simulink model "bh_SM_quad_and_PEND_ORIG"  (R2020a)
settings: Solver=ode23t  StartTime=0.0  StopTime=200  FixedStep=0.001  RelTol=1e-5  EnableMultiTasking=on
undefined symbols (not defined in the file or in its folder): K, P_elec, P_mot, P_one_prop, P_pend, P_rot, P_veh, P_veh_no_props, sigbuilder_block, X, xme_dot_0, Y, Z
libraries: fl_lib x85, nesl_utility x39, sm_lib x30, simulink_extras x15, simulink x7, fl_ps_legacy_lib x7, bh_6dof_LIBRARY x1
(part 1 of 4)
settings Model: Creator=bhorton  LastModifiedBy=bhorton
settings DataIOCC: SaveOutput=off  SignalLogging=off  DSMLogging=off  VisualizeSimOutput=off  SaveTime=off  ReturnWorkspaceOutputs=off
settings OptimizationCC: LifeSpan=inf
settings DebuggingCC: AllowSymbolicDim=off  PregeneratedLibrarySubsystemCodeDiagnostic=none  SFUnexpectedBacktrackingDiag=warning  SFNoUnconditionalDefaultTransitionDiag=warning  SFExecutionAtInitializationDiag=none  ArithmeticOperatorsInVariantConditions=warning
settings ModelReferenceCC: PropagateSignalLabelsOutOfModel=off
settings SFSimCC: SimUseLocalCustomCode=off  CustomCodeUndefinedFunction=UseInterfaceOnly
settings RTWCC: RTWUseLocalCustomCode=off
settings CodeAppCC: StateflowObjectComments=on
settings GRTTargetCC: TargetLangStandard=C89/C90 (ANSI)
settings ConfigComp: CovMetricSettings=dw  CovHtmlReporting=on  CovSaveCumulativeToWorkspaceVar=on  CovSaveSingleToWorkspaceVar=on  CovExternalEMLEnable=off
settings SimscapeCC: SimscapeNormalizeSystem=off
settings ExplorerConfigSet: InternalSimMechanicsExplorerSettings="<ExplorerConfiguration><canonicalview>default</canonicalview><AnimationSetting><BasePlaybackSpeed>1.0</BasePlaybackSpeed><PlaybackSpeedFactor>1.0</PlaybackSpeedFactor></AnimationSetting><TilePanel><TileInfo><Tiles Columns=\"2\" Count=\"2\" Rows=\"1\"><Column Weight=\"0.5\"/><Column Weight=\"0.5\"/><Row Weight=\"1\"/><Tile Height=\"1\" Width=\"1\" X=\"0\" Y=\"0\"/><Tile Height=\"1\" Width=\"1\" X=\"1\" Y=\"0\"/></Tiles></TileInfo><SceneInfo><SceneViewer><BGColor><R>0.60000002384185791</R><G>0.60000002384185791</G><B>0.60000002384185791</B></BGColor><Camera><DoPerspective>off</DoPerspective><Position><X>0.00849114839519253539</X><Y>-2.53854659515440062e-08</Y><Z>3.49084187012716951</Z></Position><Center><X>0.00849114839519253539</X><Y>-2.53854659515440062e-08</Y><Z>0.496908196154688397</Z></Center><Up><X>0</X><Y>1</Y><Z>-0</Z></Up><ViewLimDist>1</ViewLimDist><YLim>2.74755297638475904</YLim><XLim>2.06874577045440677</XLim></Camera></SceneViewer><SceneViewer><BGColor><R>0.60000002384185791</R><G>0.60000002384185791</G><B>0.60000002384185791</B></BGColor><Camera><DoPerspective>off</DoPerspective><Position><X>-0.0880664263812265952</X><Y>-3.44017982573823566</Y><Z>-0.453851828286025272</Z></Position><Center><X>0.0240437885265623319</X><Y>0.0741902828419561955</Y><Z>-0.44644297123516069</Z></Center><Up><X>-0.0156127273909268342</X><Y>-0.00160984700387389879</Y><Z>0.999876817981115718</Z></Up><ViewLimDist>1</ViewLimDist><YLim>2.91620830200649817</YLim><XLim>2.19573330974606939</XLim></Camera></SceneViewer></SceneInfo></TilePanel><MechEditorPanel><Cameras/><GfxPanelCameraMap/><VideoCreator><PlaybackSpeedRatio>1.0</PlaybackSpeedRatio><FrameRate>30</FrameRate><VideoFormat>Motion JPEG AVI</VideoFormat><FrameSize>auto</FrameSize></VideoCreator></MechEditorPanel></ExplorerConfiguration>"

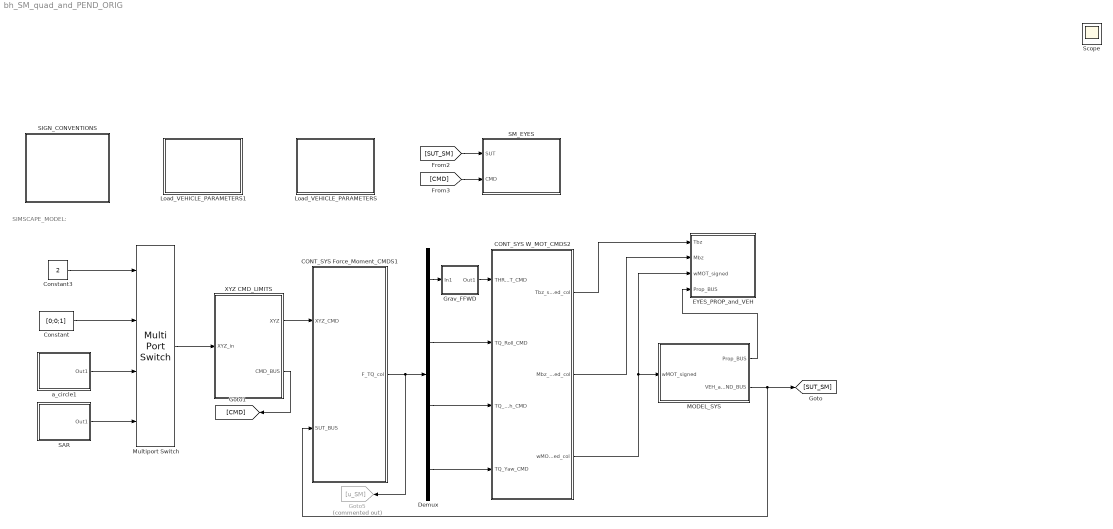
== system bh_SM_quad_and_PEND_ORIG ==
  note: SIMSCAPE_MODEL:
  CONT_SYS Force_Moment_CMDS1 : Subsystem
  CONT_SYS W_MOT_CMDS2 : Subsystem
  Constant : Constant  Value=[0;0;1]  VectorParams1D=off
  Constant3 : Constant  Value=2
  Demux : Demux
  EYES_PROP_and_VEH : Subsystem
  Goto5 : Goto  Commented=on  GotoTag=u_SM
  Grav_FFWD : Subsystem
  Load_VEHICLE_PARAMETERS : Subsystem
      settings: OpenFcn=bh_create_local_params_QP
      mask Display: disp('Double click\nto\nLOAD\nvehicle and\n PENDULUM\n parameters')
  Load_VEHICLE_PARAMETERS1 : Subsystem
      settings: AttributesFormatString=OpenFcn = %<OpenFcn>  OpenFcn=load bh_CONT_DES_RESULTS.mat
      mask Display: disp('Double click\nto\nLOAD the\nControl LAW')
  MODEL_SYS : Subsystem
  Multiport Switch : MultiPortSwitch
  SAR : Subsystem
  SIGN_CONVENTIONS : Subsystem
  SM_EYES : Subsystem
      mask Display: image('bh_PIC_SCOPE.jpg');
  XYZ CMD_LIMITS : Subsystem
  a_circle1 : Subsystem
  Scope : Scope
  wires:
  [SUT_SM] -> SM_EYES/1(SUT)
  [CMD] -> SM_EYES/2(CMD)
  XYZ CMD_LIMITS/1(XYZ) -> CONT_SYS Force_Moment_CMDS1/1(XYZ_CMD)
  XYZ CMD_LIMITS/2(CMD_BUS) -> [CMD]
  MODEL_SYS/2(VEH_and_PEND_BUS) -> CONT_SYS Force_Moment_CMDS1/2(SUT_BUS), [SUT_SM]
  Demux/1 -> Grav_FFWD/1(In1)
  Demux/2 -> CONT_SYS W_MOT_CMDS2/2(TQ_Roll_CMD)
  Demux/3 -> CONT_SYS W_MOT_CMDS2/3(TQ_Pitch_CMD)
  Demux/4 -> CONT_SYS W_MOT_CMDS2/4(TQ_Yaw_CMD)
  Grav_FFWD/1(Out1) -> CONT_SYS W_MOT_CMDS2/1(THRUST_CMD)
  Constant/1 -> Multiport Switch/2
  Constant3/1 -> Multiport Switch/1
  SAR/1(Out1) -> Multiport Switch/4
  a_circle1/1(Out1) -> Multiport Switch/3
  Multiport Switch/1 -> XYZ CMD_LIMITS/1(XYZ_in)
  MODEL_SYS/1(Prop_BUS) -> EYES_PROP_and_VEH/4(Prop_BUS)
  CONT_SYS Force_Moment_CMDS1/1(F_TQ_col) -> Demux/1, Goto5/1
  CONT_SYS W_MOT_CMDS2/3(wMOT_signed_col) -> EYES_PROP_and_VEH/3(wMOT_signed), MODEL_SYS/1(wMOT_signed)
  CONT_SYS W_MOT_CMDS2/2(Mbz_signed_col) -> EYES_PROP_and_VEH/2(Mbz)
  CONT_SYS W_MOT_CMDS2/1(Tbz_signed_col) -> EYES_PROP_and_VEH/1(Tbz)

== system bh_SM_quad_and_PEND_ORIG/CONT_SYS Force_Moment_CMDS1 ==
  XYZ_CMD : Inport
  SUT_BUS : Inport  Port=2
  Bus Selector : BusSelector  OutputSignals=Xe
  Bus Selector1 : BusSelector  OutputSignals=DOT_phi_theta_psi,Ve,pend_bus.DOT_phi_theta_psi,phi_theta_psi,Xe,pend_bus.phi_theta_psi
  Constant1 : Constant  Value=[0;0;0]  VectorParams1D=off
  Constant2 : Constant  Value=K  VectorParams1D=off
  Constant3 : Constant  Commented=on  Value=P_veh.mass
  Gain : Gain  Commented=on  Gain=9.81
  Gain1 : Gain  Gain=-1
  Integrator : Integrator  InitialConditionSource=external
  Mux : Mux  Inputs=7
  Product1 : Product  Multiplication=Matrix(*)
  Reshape{,1..7} (8 alike) : Reshape  OutputDimensionality=Column vector (2-D)
  Sum : Sum  Inputs=|+-
  F_TQ_col : Outport  VectorParamsAs1DForOutWhenUnconnected=off
  wires:
  SUT_BUS/1 -> [SUT], Bus Selector/1
  Constant3/1 -> Gain/1
  Constant1/1 -> Integrator/2
  Integrator/1 -> Reshape/1
  Reshape/1 -> Mux/7
  XYZ_CMD/1 -> Sum/1
  Sum/1 -> Integrator/1
  Bus Selector/1 -> Sum/2  "<Xe>"
  [SUT] -> Bus Selector1/1
  Bus Selector1/1 -> Reshape1/1  "<DOT_phi_theta_psi>"
  Bus Selector1/2 -> Reshape2/1  "<Ve>"
  Bus Selector1/4 -> Reshape3/1  "<phi_theta_psi>"
  Bus Selector1/5 -> Reshape4/1  "<Xe>"
  Constant2/1 -> Gain1/1
  Gain1/1 -> Product1/1
  Mux/1 -> Product1/2
  Product1/1 -> Reshape5/1
  Reshape5/1 -> F_TQ_col/1
  Bus Selector1/6 -> Reshape6/1  "<phi_theta_psi>"
  Bus Selector1/3 -> Reshape7/1  "<DOT_phi_theta_psi>"
  Reshape1/1 -> Mux/1
  Reshape2/1 -> Mux/2
  Reshape7/1 -> Mux/3
  Reshape3/1 -> Mux/4
  Reshape4/1 -> Mux/5
  Reshape6/1 -> Mux/6

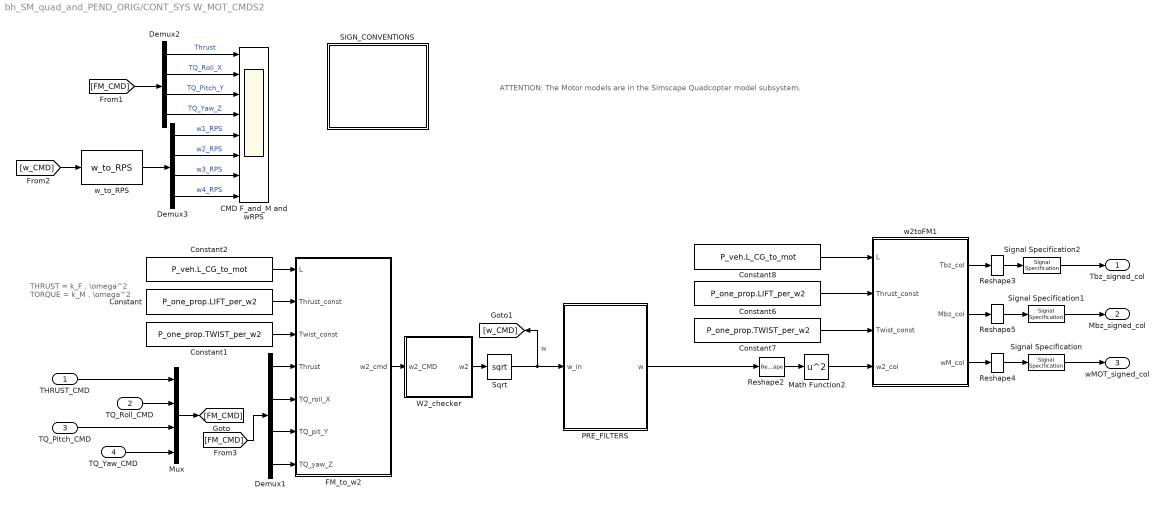
== system bh_SM_quad_and_PEND_ORIG/CONT_SYS W_MOT_CMDS2 ==
  note: ATTENTION:
      | The Motor models are in the Simscape
      | Quadcopter model subsystem.
  note: THRUST = k_F . \omega^2
      |
      | TORQUE = k_M . \omega^2
  THRUST_CMD : Inport
  TQ_Roll_CMD : Inport  Port=2
  TQ_Pitch_CMD : Inport  Port=3
  TQ_Yaw_CMD : Inport  Port=4
  CMD F_and_M and wRPS : Scope  NumInputPorts=8
  Constant : Constant  Value=P_one_prop.LIFT_per_w2
  Constant1 : Constant  Value=P_one_prop.TWIST_per_w2
  Constant2 : Constant  Value=P_veh.L_CG_to_mot
  Constant6 : Constant  Value=P_one_prop.LIFT_per_w2
  Constant7 : Constant  Value=P_one_prop.TWIST_per_w2
  Constant8 : Constant  Value=P_veh.L_CG_to_mot
  Demux1 : Demux
  Demux2 : Demux
  Demux3 : Demux
  FM_to_w2 : MATLAB Function  TreatAsAtomicUnit=on
  Math Function2 : Math  Operator=square  SignedPower=on  SaturateOnIntegerOverflow=on
  Mux : Mux
  PRE_FILTERS : Subsystem
  Reshape{2..5} (4 alike) : Reshape  OutputDimensionality=Column vector (2-D)
  SIGN_CONVENTIONS : Subsystem
  Signal Specification : SignalSpecification  Dimensions=[4,1]
  Signal Specification1 : SignalSpecification  Dimensions=[4,1]
  Signal Specification2 : SignalSpecification  Dimensions=[4,1]
  Sqrt : Sqrt  SaturateOnIntegerOverflow=on
  W2_checker : Subsystem
  w2toFM1 : MATLAB Function  TreatAsAtomicUnit=on
  w_to_RPS : bh_6dof_LIBRARY/MODELS/w_to_RPS  SystemSampleTime=-1  Latency=0  AutoFrameSizeCalculation=off
  Tbz_signed_col : Outport  VectorParamsAs1DForOutWhenUnconnected=off
  Mbz_signed_col : Outport  Port=2  VectorParamsAs1DForOutWhenUnconnected=off
  wMOT_signed_col : Outport  Port=3  VectorParamsAs1DForOutWhenUnconnected=off
  wires:
  Constant1/1 -> FM_to_w2/3(Twist_const)
  Constant/1 -> FM_to_w2/2(Thrust_const)
  Constant2/1 -> FM_to_w2/1(L)
  Sqrt/1 -> PRE_FILTERS/1(w_in), [w_CMD]  "w"
  W2_checker/1(w2) -> Sqrt/1
  Demux1/1 -> FM_to_w2/4(Thrust)
  Demux1/2 -> FM_to_w2/5(TQ_roll_X)
  Demux1/3 -> FM_to_w2/6(TQ_pit_Y)
  Demux1/4 -> FM_to_w2/7(TQ_yaw_Z)
  THRUST_CMD/1 -> Mux/1
  TQ_Roll_CMD/1 -> Mux/2
  TQ_Pitch_CMD/1 -> Mux/3
  TQ_Yaw_CMD/1 -> Mux/4
  Mux/1 -> [FM_CMD]
  [FM_CMD] -> Demux1/1
  Demux2/1 -> CMD F_and_M and wRPS/1  "Thrust"
  Demux2/2 -> CMD F_and_M and wRPS/2  "TQ_Roll_X"
  Demux2/3 -> CMD F_and_M and wRPS/3  "TQ_Pitch_Y"
  Demux2/4 -> CMD F_and_M and wRPS/4  "TQ_Yaw_Z"
  Demux3/2 -> CMD F_and_M and wRPS/6  "w2_RPS"
  Demux3/1 -> CMD F_and_M and wRPS/5  "w1_RPS"
  Demux3/4 -> CMD F_and_M and wRPS/8  "w4_RPS"
  Demux3/3 -> CMD F_and_M and wRPS/7  "w3_RPS"
  [FM_CMD] -> Demux2/1
  w_to_RPS/1 -> Demux3/1
  [w_CMD] -> w_to_RPS/1
  Reshape2/1 -> Math Function2/1
  Math Function2/1 -> w2toFM1/4(w2_col)
  Constant7/1 -> w2toFM1/3(Twist_const)
  Constant6/1 -> w2toFM1/2(Thrust_const)
  Constant8/1 -> w2toFM1/1(L)
  w2toFM1/2(Mbz_col) -> Reshape5/1
  w2toFM1/1(Tbz_col) -> Reshape3/1
  w2toFM1/3(wM_col) -> Reshape4/1
  Reshape3/1 -> Signal Specification2/1
  Reshape5/1 -> Signal Specification1/1
  Reshape4/1 -> Signal Specification/1
  Signal Specification2/1 -> Tbz_signed_col/1
  Signal Specification1/1 -> Mbz_signed_col/1
  Signal Specification/1 -> wMOT_signed_col/1
  FM_to_w2/1(w2_cmd) -> W2_checker/1(w2_CMD)
  PRE_FILTERS/1(w) -> Reshape2/1

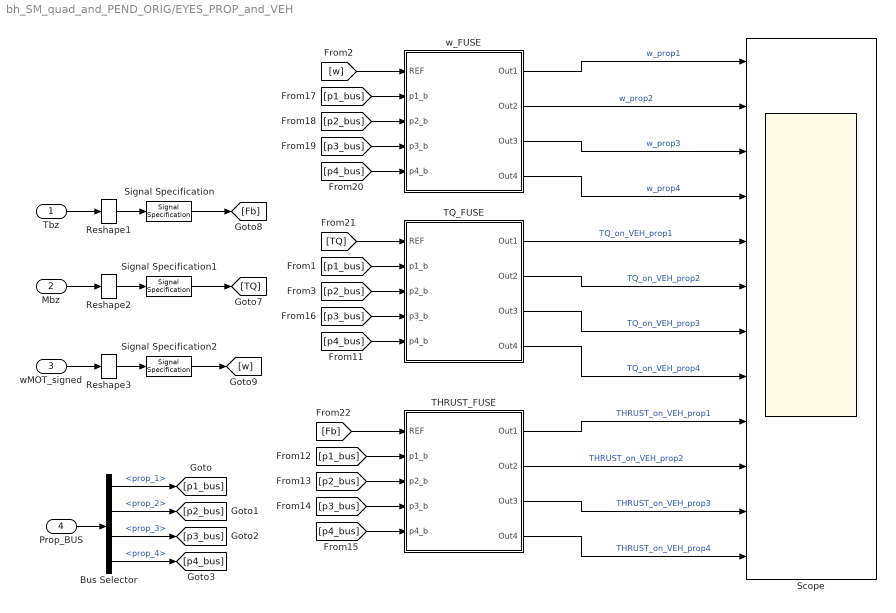
== system bh_SM_quad_and_PEND_ORIG/EYES_PROP_and_VEH ==
  Tbz : Inport
  Mbz : Inport  Port=2
  wMOT_signed : Inport  Port=3
  Prop_BUS : Inport  Port=4
  Bus Selector : BusSelector  OutputSignals=prop_1,prop_2,prop_3,prop_4
  Reshape1 : Reshape  OutputDimensionality=Column vector (2-D)
  Reshape2 : Reshape  OutputDimensionality=Column vector (2-D)
  Reshape3 : Reshape  OutputDimensionality=Column vector (2-D)
  Scope : Scope  NumInputPorts=12
  Signal Specification : SignalSpecification  Dimensions=[4,1]
  Signal Specification1 : SignalSpecification  Dimensions=[4,1]
  Signal Specification2 : SignalSpecification  Dimensions=[4,1]
  THRUST_FUSE : Subsystem
  TQ_FUSE : Subsystem
  w_FUSE : Subsystem
  wires:
  Reshape2/1 -> Signal Specification1/1
  Reshape1/1 -> Signal Specification/1
  Tbz/1 -> Reshape1/1
  Signal Specification1/1 -> [TQ]
  Mbz/1 -> Reshape2/1
  Prop_BUS/1 -> Bus Selector/1
  [p3_bus] -> w_FUSE/4(p3_b)
  [p3_bus] -> THRUST_FUSE/4(p3_b)
  [p4_bus] -> w_FUSE/5(p4_b)
  w_FUSE/2(Out2) -> Scope/2  "w_prop2"
  [p2_bus] -> w_FUSE/3(p2_b)
  THRUST_FUSE/2(Out2) -> Scope/10  "THRUST_on_VEH_prop2"
  THRUST_FUSE/1(Out1) -> Scope/9  "THRUST_on_VEH_prop1"
  [p2_bus] -> TQ_FUSE/3(p2_b)
  THRUST_FUSE/4(Out4) -> Scope/12  "THRUST_on_VEH_prop4"
  TQ_FUSE/2(Out2) -> Scope/6  "TQ_on_VEH_prop2"
  TQ_FUSE/3(Out3) -> Scope/7  "TQ_on_VEH_prop3"
  [p3_bus] -> TQ_FUSE/4(p3_b)
  TQ_FUSE/4(Out4) -> Scope/8  "TQ_on_VEH_prop4"
  TQ_FUSE/1(Out1) -> Scope/5  "TQ_on_VEH_prop1"
  [w] -> w_FUSE/1(REF)
  w_FUSE/3(Out3) -> Scope/3  "w_prop3"
  w_FUSE/4(Out4) -> Scope/4  "w_prop4"
  [p4_bus] -> THRUST_FUSE/5(p4_b)
  THRUST_FUSE/3(Out3) -> Scope/11  "THRUST_on_VEH_prop3"
  [Fb] -> THRUST_FUSE/1(REF)
  w_FUSE/1(Out1) -> Scope/1  "w_prop1"
  [p2_bus] -> THRUST_FUSE/3(p2_b)
  [p1_bus] -> THRUST_FUSE/2(p1_b)
  [TQ] -> TQ_FUSE/1(REF)
  [p4_bus] -> TQ_FUSE/5(p4_b)
  [p1_bus] -> w_FUSE/2(p1_b)
  [p1_bus] -> TQ_FUSE/2(p1_b)
  Signal Specification/1 -> [Fb]
  wMOT_signed/1 -> Reshape3/1
  Reshape3/1 -> Signal Specification2/1
  Signal Specification2/1 -> [w]
  Bus Selector/4 -> [p4_bus]  "<prop_4>"
  Bus Selector/3 -> [p3_bus]  "<prop_3>"
  Bus Selector/2 -> [p2_bus]  "<prop_2>"
  Bus Selector/1 -> [p1_bus]  "<prop_1>"

== system bh_SM_quad_and_PEND_ORIG/Grav_FFWD ==
  In1 : Inport
  Constant3 : Constant  Value=P_veh.mass + P_pend.mass
  Gain : Gain  Gain=9.81
  Sum : Sum  Inputs=++|
  Out1 : Outport  VectorParamsAs1DForOutWhenUnconnected=off
  wires:
  Gain/1 -> Sum/1
  Constant3/1 -> Gain/1
  Sum/1 -> Out1/1
  In1/1 -> Sum/2

== system bh_SM_quad_and_PEND_ORIG/Load_VEHICLE_PARAMETERS ==

== system bh_SM_quad_and_PEND_ORIG/Load_VEHICLE_PARAMETERS1 ==

== system bh_SM_quad_and_PEND_ORIG/MODEL_SYS ==
  wMOT_signed : Inport
  Bus Creator : BusCreator  Inputs=10
  Reshape3 : Reshape  OutputDimensionality=Column vector (2-D)
  SIGN_CONVENTIONS : Subsystem
  Signal Specification2 : SignalSpecification  Dimensions=[4,1]
  WAY_POINT_PLOTS : sm_lib/Curves and Surfaces/Spline  GraphicAmbientColor=[0.15 0.15 0.15 1.0]  GraphicDiffuseColor=[0.0 1.0 0.2]  DataPoints=XYZ_circ_mat  DataPointsUnits=m  GraphicEmissiveColor=[0.0 0.0 0.0 1.0]  EndConditionType=Natural  MarkerShape=Cube  MarkerSize=10  GraphicType=FromGeometry  GraphicOpacity=1.0  GraphicShininess=75  GraphicSpecularColor=[0.5 0.5 0.5 1.0]  GraphicVisPropType=SimpleVisualProperties
  bh_6DOF (Simscape) : Subsystem  mask(bh_6DOF EoM (Body Axis)){air_inertia_0=P_veh_no_props.I, air_mass_0=P_veh_no_props.mass, xme_0=P_veh_no_props.Xe_init, Vm_0=P_veh_no_props.Vb_init, pm_0=P_veh_no_props.wb_init, eul_0=P_veh_no_props.eul_init, prop_Imat=P_rot.I, prop_mass=P_rot.mass, prop_CG_L=P_veh_no_props.L_CG_to_mot, prop_CG_H=P_veh_no_props.H_CG_to_mot, g_const=9.80665, I_pend=P_pend.I, m_pend=P_pend.mass, L_pend_XYZ=P_pend.L_xyz, T_pend_XYZ=P_pend.T_xyz, eul_0_pend=P_pend.eul_loc_vec}
      mask prompts: air_inertia_0 "Airframe Inertia, [kg.m^2]"; air_mass_0 "Airframe Mass, [kg]"; xme_0 "Initial position in inertial axes [Xe,Ye,Ze], [m]"; Vm_0 "Initial velocity in body axes [U,v,w], [m/sec]"; pm_0 "Initial body rotation rates [p,q,r], [rad/sec]"; eul_0 "Initial Euler orientation [yaw, pitch, roll], [rad]"; prop_Imat "Propeller Assembly Inertia [kg*m^2]"; prop_mass "Propeller Assembly Mass [kg]"; prop_CG_L "Airframe CG to Prop CG distance - L [m]"; prop_CG_H "Airframe CG to Prop CG distance - H [m]"; g_const "Gravity constant [m/sec^2]"; I_pend "Inertia of Pendulum through it's CoM [kg.m^2]"; m_pend "Mass of pendulum [kg]"; L_pend_XYZ "Lengths of Pendulum (X,Y,Z)  [m]"; T_pend_XYZ "Position of Spherical joint T(X,Y,Z) [m]"; eul_0_pend "Initial Euler orientation [yaw, pitch, roll], [rad]"
      mask init:
      | [  Iair_xx_yy_zz,  ...
      |    Iair_yz_zx_xy,  ...
      |    Iprop_xx_yy_zz, ...
      |    Iprop_yz_zx_xy, ...
      |    xme_dot_0,      ...
      |    eul_dot_0  ] =  ...
      |    bh_func_for_lagr_mask_init( air_inertia_0,  ... 
      |                                prop_Imat,      ...
      |                                Vm_0,           ...
      |                                pm_0,           ...
      |                                eul_0); 
      |                            
      |   Ipend_xx_yy_zz = [I_pend(1,1), I_pend(2,2), I_pend(3,3)];  
      |   Ipend_yz_zx_xy = [I_pend(2,3), I_pend(3,1), I_pend(1,2)];
      mask DialogControl DescTextVar Prompt: Implementation of a 6-DOF rigid body equations of motion.
      mask DialogControl Control16 Prompt: Euler angles are used to describe angular pose.
      mask DialogControl Container4 Prompt: Airframe
      mask DialogControl Control11 Prompt: ATTENTION:  note the order of the angles in the list above.
      mask DialogControl Control12 Prompt: This is DIFFERENT to the order used in the Aerospace blockset.
      mask DialogControl Container19 Prompt: Propeller
      mask DialogControl Container13 Prompt: ENVIRONMENT
      mask DialogControl Control42 Prompt: NOTE:  the Gravity constant should be a POSITIVE number, eg: 9.81
      mask DialogControl Container14 Prompt: Pendulum
      mask DialogControl Control50 Prompt: Position of Spherical joint relative to airframe CoM:
      mask DialogControl Control41 Prompt: Define the Euler angles of {P}-frame relative to {V}-frame.  The rotation
      mask DialogControl Control45 Prompt: sequence is Z-Y-X  as [Phi,Theta,Psi]
      mask DialogControl Container20 Prompt: Geometry
      mask DialogControl Container21 Prompt: Axes
      mask DialogControl Container6 Prompt: DOC
      mask DialogControl Control6 Prompt: In this EULER angle implementation we define the
      mask DialogControl Control7 Prompt: following sequence that rotates a G-frame
      mask DialogControl Control8 Prompt: into a B-frame:
      mask DialogControl Control9_copy Prompt: 1.)  R1Z  : a local rotation about the Z axis by phi, (YAW)
      mask DialogControl Control9_copy_copy Prompt: 2.)  R2Y  : a local rotation about the Y axis by theta, (PITCH)
      mask DialogControl Control17 Prompt: 3.)  R3X  : a local rotation about the X axis by psi, (ROLL)
      mask DialogControl Container16 Prompt: PASSIVE rotation sequence
      mask DialogControl Control22 Prompt: The co-ordinate transformation that converts the components of a
      mask DialogControl Control23 Prompt: G-frame vector into its components in the B-frame, is:
      mask DialogControl Control24 Prompt: vb = pR3X(psi) * pR2Y(theta) * pR1Z(phi) * vg
      mask DialogControl Control25 Prompt: vb = bRg * vg
      mask DialogControl Control53 Prompt: You can READ more about PASSIVE rotations, HERE.
      mask DialogControl Control53 Callback: winopen('CONCEPT_PASSIVE_rotations.pdf')
      mask DialogControl Container22 Prompt: ACTIVE rotation sequence
      mask DialogControl Control26 Prompt: To actively reposition (ie: rotate) a B-frame that is initially coincident
      mask DialogControl Control27 Prompt: with the inertial G-frame, into a new pose, we would:
      mask DialogControl Control28 Prompt: vg = inv(pR1Z(phi)) * inv(pR2Y(theta)) * inv(pR3X(psi)) * vb
      mask DialogControl Control30 Prompt: If we define:    aR( ) == inv( pR()  ),  then we can write the above as:
      mask DialogControl Control32 Prompt: vg = aR1Z(phi) * aR2Y(theta) * aR3(psi) * vb
      mask DialogControl Control40 Prompt: You can READ more about ACTIVE rotations, HERE.
      mask DialogControl Control40 Callback: winopen('CONCEPT_ACTIVE_rotations.pdf')
      mask Display:
      | %port_label('input',1,'{{Tbz_{mot}} (N)}','texmode','on');
      | %port_label('input',2,'{{Mbz_{mot}} (N-m)}','texmode','on');
      | port_label('input',1,'{{\omega_{mot}} (rad/sec)}','texmode','on');
      | port_label('output',1,'{V_e (m/s)}','texmode','on');
      | port_label('output',2,'{X_e (m)}','texmode','on');
      | port_label('output',3,'{\Phi_{Z1} \theta_{Y2} \Psi_{X3} (rad)}','texmode','on');
      | port_label('output',4,'{DCM bRg }','texmode','on');
      | port_label('output',5,'{V_b (m/s)}','texmode','on');
      | port_label('output',6,'{{\omega_b (rad/s)}}','texmode','on');
      | port_label('output',7,'{{d\omega_b/dt}}','texmode','on');
      | port_label('output',8,'{A_b (m/s^2)}','texmode','on');
      | port_label('output',9,'{d\Phi_{Z1} d\theta_{Y2} d\Psi_{X3} (rad/sec)}','texmode','on');
      | port_label('output',10, 'Pend_BUS');
      | port_label('output',11, 'Prop_BUS');
      | text(0.5,0.7248,'Simscape \nBody\nEuler Angles \n\n\n\n\n PENDULUM','horizontalAlignment','center')
  Prop_BUS : Outport  VectorParamsAs1DForOutWhenUnconnected=off
  VEH_and_PEND_BUS : Outport  Port=2  OutDataTypeStr=Bus: VEH_AND_PEND_BUS  VectorParamsAs1DForOutWhenUnconnected=off
  wires:
  Signal Specification2/1 -> bh_6DOF (Simscape)/1(wMOT)
  bh_6DOF (Simscape)/4(bRg (DCM)) -> Bus Creator/4  "DCM_bRg"
  bh_6DOF (Simscape)/5(Vb) -> Bus Creator/5  "Vb"
  bh_6DOF (Simscape)/6(p,q,r) -> Bus Creator/6  "wb_pqr"
  bh_6DOF (Simscape)/8(Ab) -> Bus Creator/8  "Ab"
  Bus Creator/1 -> VEH_and_PEND_BUS/1
  bh_6DOF (Simscape)/7(pdot,qdot,rdot) -> Bus Creator/7  "DOT_wb"
  wMOT_signed/1 -> Reshape3/1
  bh_6DOF (Simscape)/9(Euler_rates) -> Bus Creator/9  "DOT_phi_theta_psi"
  bh_6DOF (Simscape)/3(Euler) -> Bus Creator/3  "phi_theta_psi"
  Reshape3/1 -> Signal Specification2/1
  bh_6DOF (Simscape)/1(Ve) -> Bus Creator/1  "Ve"
  bh_6DOF (Simscape)/2(Xe) -> Bus Creator/2  "Xe"
  bh_6DOF (Simscape)/10(pend_bus) -> Bus Creator/10  "pend_bus"
  bh_6DOF (Simscape)/11(Prop_Bus) -> [Prop_BUS]
  [Prop_BUS] -> Prop_BUS/1
  connections:
  WAY_POINT_PLOTS/LConn1 -- bh_6DOF (Simscape)/LConn1

== system bh_SM_quad_and_PEND_ORIG/SAR ==
  Mux : Mux  Inputs=3
  Selector : Selector  InputPortWidth=3  IndexOptions=Index vector (dialog)  Indices=[2 3 1]  OutputSizes=1
  XYZ_CMDS : Subsystem  Tag=STV Subsys  LoadFcn=sigbuilder_block('load');  StartFcn=sigbuilder_block('start');  StopFcn=sigbuilder_block('stop');  ClipboardFcn=sigbuilder_block('clipboard');  mask(Sigbuilder block){tuvar=[0:10]}
      mask help: Simulink:masks:SigbuilderBlock_MD
      mask init:
      | if ~strcmp(get_param(bdroot(gcbh),'SimulationStatus'),'stopped') tuvar = sigbuilder_block('maskInit'); end
      settings: CopyFcn=sigbuilder_block('copy');  DeleteFcn=sigbuilder_block('delete');  ModelCloseFcn=sigbuilder_block('modelClose');  PreSaveFcn=sigbuilder_block('preSave');  PauseFcn=sigbuilder_block('pause');  ContinueFcn=sigbuilder_block('continue');  NameChangeFcn=sigbuilder_block('namechange');  OpenFcn=sigbuilder_block('open',[189 32.25 551.25 400.5 ]);  CloseFcn=sigbuilder_block('close');
      mask Display: plot(0, 0, 100, 100,[2, 2, 32, 32, 2], [68, 8, 8, 68, 68],[32, 2], [38, 38], [32, 19, 2],[53, 60, 44], [32, 17, 17, 2],[16, 16, 31, 31]);txt = getActiveGroup(gcbh);text(2, 100, txt,'verticalAlignment', 'top');
  Out1 : Outport  VectorParamsAs1DForOutWhenUnconnected=off
  wires:
  XYZ_CMDS/3(Y) -> Mux/3
  XYZ_CMDS/1(Z) -> Mux/1
  XYZ_CMDS/2(X) -> Mux/2
  Mux/1 -> Selector/1
  Selector/1 -> Out1/1

== system bh_SM_quad_and_PEND_ORIG/SIGN_CONVENTIONS ==

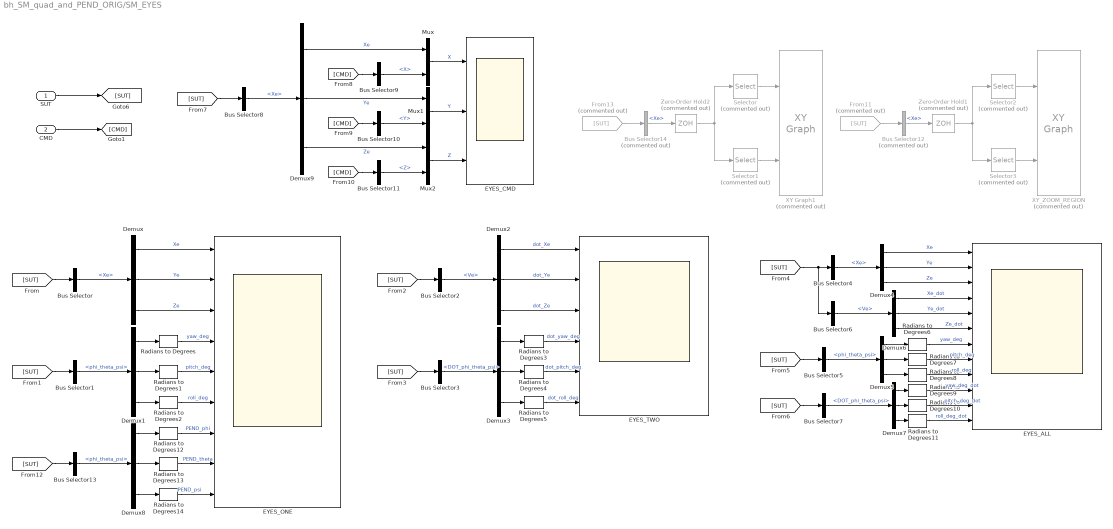
== system bh_SM_quad_and_PEND_ORIG/SM_EYES ==
  SUT : Inport
  CMD : Inport  Port=2
  Bus Selector : BusSelector  OutputSignals=Xe
  Bus Selector1 : BusSelector  OutputSignals=phi_theta_psi
  Bus Selector10 : BusSelector  OutputSignals=Y
  Bus Selector11 : BusSelector  OutputSignals=Z
  Bus Selector12 : BusSelector  Commented=on  OutputSignals=Xe
  Bus Selector13 : BusSelector  OutputSignals=pend_bus.phi_theta_psi
  Bus Selector14 : BusSelector  Commented=on  OutputSignals=Xe
  Bus Selector2 : BusSelector  OutputSignals=Ve
  Bus Selector3 : BusSelector  OutputSignals=DOT_phi_theta_psi
  Bus Selector4 : BusSelector  OutputSignals=Xe
  Bus Selector5 : BusSelector  OutputSignals=phi_theta_psi
  Bus Selector6 : BusSelector  OutputSignals=Ve
  Bus Selector7 : BusSelector  OutputSignals=DOT_phi_theta_psi
  Bus Selector8 : BusSelector  OutputSignals=Xe
  Bus Selector9 : BusSelector  OutputSignals=X
  Demux{,1..9} (10 alike) : Demux  Outputs=3
  EYES_ALL : Scope  NumInputPorts=12
  EYES_CMD : Scope  NumInputPorts=3
  EYES_ONE : Scope  NumInputPorts=9
  EYES_TWO : Scope  NumInputPorts=6
  From11 : From  Commented=on  GotoTag=SUT
  From13 : From  Commented=on  GotoTag=SUT
  Mux : Mux  Inputs=2
  Mux1 : Mux  Inputs=2
  Mux2 : Mux  Inputs=2
  Radians to Degrees{,1..14} (15 alike) : simulink_extras/Transformations/Radians to Degrees
  Selector : Selector  Commented=on  InputPortWidth=3  IndexOptions=Index vector (dialog)  Indices=1  OutputSizes=1
  Selector1 : Selector  Commented=on  InputPortWidth=3  IndexOptions=Index vector (dialog)  Indices=2  OutputSizes=1
  Selector2 : Selector  Commented=on  InputPortWidth=3  IndexOptions=Index vector (dialog)  Indices=1  OutputSizes=1
  Selector3 : Selector  Commented=on  InputPortWidth=3  IndexOptions=Index vector (dialog)  Indices=2  OutputSizes=1
  XY Graph1 : simulink/Sinks/XY Graph  Commented=on  xmin=-1  xmax=30  ymin=-1  ymax=35  st=-1
  XY_ZOOM_REGION : simulink/Sinks/XY Graph  Commented=on  xmin=-3  xmax=3  ymin=-3  ymax=3  st=-1
  Zero-Order Hold1 : ZeroOrderHold  Commented=on  SampleTime=0.1
  Zero-Order Hold2 : ZeroOrderHold  Commented=on  SampleTime=0.1
  wires:
  SUT/1 -> [SUT]
  [SUT] -> Bus Selector/1
  Demux/2 -> EYES_ONE/2  "Ye"
  Demux/3 -> EYES_ONE/3  "Ze"
  Demux/1 -> EYES_ONE/1  "Xe"
  Bus Selector/1 -> Demux/1  "<Xe>"
  Bus Selector1/1 -> Demux1/1  "<phi_theta_psi>"
  [SUT] -> Bus Selector1/1
  Demux1/1 -> Radians to Degrees/1
  Radians to Degrees/1 -> EYES_ONE/4  "yaw_deg"
  Radians to Degrees1/1 -> EYES_ONE/5  "pitch_deg"
  Radians to Degrees2/1 -> EYES_ONE/6  "roll_deg"
  Demux1/3 -> Radians to Degrees2/1
  Demux1/2 -> Radians to Degrees1/1
  [SUT] -> Bus Selector2/1
  Demux2/2 -> EYES_TWO/2  "dot_Ye"
  Demux2/3 -> EYES_TWO/3  "dot_Ze"
  Demux2/1 -> EYES_TWO/1  "dot_Xe"
  Bus Selector2/1 -> Demux2/1  "<Ve>"
  Bus Selector3/1 -> Demux3/1  "<DOT_phi_theta_psi>"
  [SUT] -> Bus Selector3/1
  Demux3/1 -> Radians to Degrees3/1
  Radians to Degrees3/1 -> EYES_TWO/4  "dot_yaw_deg"
  Radians to Degrees4/1 -> EYES_TWO/5  "dot_pitch_deg"
  Radians to Degrees5/1 -> EYES_TWO/6  "dot_roll_deg"
  Demux3/3 -> Radians to Degrees5/1
  Demux3/2 -> Radians to Degrees4/1
  [SUT] -> Bus Selector6/1, Bus Selector4/1
  Demux4/2 -> EYES_ALL/2  "Ye"
  Demux4/3 -> EYES_ALL/3  "Ze"
  Demux4/1 -> EYES_ALL/1  "Xe"
  Bus Selector4/1 -> Demux4/1  "<Xe>"
  Bus Selector5/1 -> Demux5/1  "<phi_theta_psi>"
  [SUT] -> Bus Selector5/1
  Demux5/1 -> Radians to Degrees6/1
  Demux6/1 -> EYES_ALL/4  "Xe_dot"
  Demux6/2 -> EYES_ALL/5  "Ye_dot"
  Demux6/3 -> EYES_ALL/6  "Ze_dot"
  Demux5/3 -> Radians to Degrees8/1
  Demux5/2 -> Radians to Degrees7/1
  Bus Selector6/1 -> Demux6/1  "<Ve>"
  Radians to Degrees6/1 -> EYES_ALL/7  "yaw_deg"
  Radians to Degrees7/1 -> EYES_ALL/8  "pitch_deg"
  Radians to Degrees8/1 -> EYES_ALL/9  "roll_deg"
  Bus Selector7/1 -> Demux7/1  "<DOT_phi_theta_psi>"
  [SUT] -> Bus Selector7/1
  Demux7/1 -> Radians to Degrees9/1
  Demux7/2 -> Radians to Degrees10/1
  Demux7/3 -> Radians to Degrees11/1
  Radians to Degrees9/1 -> EYES_ALL/10  "yaw_deg_dot"
  Radians to Degrees10/1 -> EYES_ALL/11  "pitch_deg_dot"
  Radians to Degrees11/1 -> EYES_ALL/12  "roll_deg_dot"
  CMD/1 -> [CMD]
  [SUT] -> Bus Selector8/1
  Demux9/2 -> Mux1/1  "Ye"
  Demux9/1 -> Mux/1  "Xe"
  Bus Selector8/1 -> Demux9/1  "<Xe>"
  Mux/1 -> EYES_CMD/1  "X"
  Mux1/1 -> EYES_CMD/2  "Y"
  Mux2/1 -> EYES_CMD/3  "Z"
  Demux9/3 -> Mux2/1  "Ze"
  [CMD] -> Bus Selector9/1
  Bus Selector9/1 -> Mux/2  "<X>"
  [CMD] -> Bus Selector10/1
  Bus Selector10/1 -> Mux1/2  "<Y>"
  [CMD] -> Bus Selector11/1
  Bus Selector11/1 -> Mux2/2  "<Z>"
  From13/1 -> Bus Selector14/1
  Bus Selector14/1 -> Zero-Order Hold2/1  "<Xe>"
  Zero-Order Hold2/1 -> Selector1/1, Selector/1
  Selector1/1 -> XY Graph1/2
  Selector/1 -> XY Graph1/1
  From11/1 -> Bus Selector12/1
  Zero-Order Hold1/1 -> Selector3/1, Selector2/1
  Selector3/1 -> XY_ZOOM_REGION/2
  Selector2/1 -> XY_ZOOM_REGION/1
  Bus Selector12/1 -> Zero-Order Hold1/1  "<Xe>"
  [SUT] -> Bus Selector13/1
  Bus Selector13/1 -> Demux8/1  "<phi_theta_psi>"
  Demux8/3 -> Radians to Degrees14/1
  Demux8/2 -> Radians to Degrees13/1
  Demux8/1 -> Radians to Degrees12/1
  Radians to Degrees12/1 -> EYES_ONE/7  "PEND_phi"
  Radians to Degrees13/1 -> EYES_ONE/8  "PEND_theta"
  Radians to Degrees14/1 -> EYES_ONE/9  "PEND_psi"

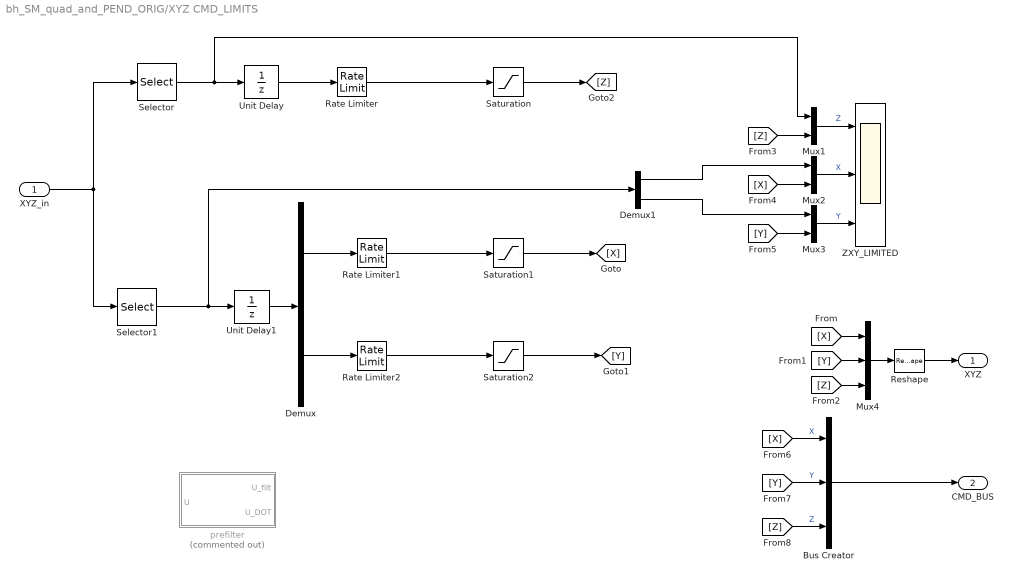
== system bh_SM_quad_and_PEND_ORIG/XYZ CMD_LIMITS ==
  XYZ_in : Inport
  Bus Creator : BusCreator  Inputs=3
  Demux : Demux  Outputs=2
  Demux1 : Demux  Outputs=2
  Mux1 : Mux  Inputs=2
  Mux2 : Mux  Inputs=2
  Mux3 : Mux  Inputs=2
  Mux4 : Mux  Inputs=3
  Rate Limiter : RateLimiter  RisingSlewLimit=2  FallingSlewLimit=-2
      settings: AttributesFormatString=|
      | Rising_rate = %<RisingSlewLimit>
      | Falling_rate = %<FallingSlewLimit>
  Rate Limiter1 : RateLimiter  RisingSlewLimit=3  FallingSlewLimit=-3
      settings: AttributesFormatString=|
      | Rising_rate = %<RisingSlewLimit>
      | Falling_rate = %<FallingSlewLimit>
  Rate Limiter2 : RateLimiter  RisingSlewLimit=3  FallingSlewLimit=-3
      settings: AttributesFormatString=|
      | Rising_rate = %<RisingSlewLimit>
      | Falling_rate = %<FallingSlewLimit>
  Reshape : Reshape  OutputDimensionality=Column vector (2-D)
  Saturation : Saturate  UpperLimit=500  LowerLimit=0
      settings: AttributesFormatString=|
      | MAX =    %<UpperLimit>
      | MIN = %<LowerLimit>
  Saturation1 : Saturate  UpperLimit=500  LowerLimit=-500
      settings: AttributesFormatString=|
      | MAX =    %<UpperLimit>
      | MIN = %<LowerLimit>
  Saturation2 : Saturate  UpperLimit=500  LowerLimit=-500
      settings: AttributesFormatString=|
      | MAX =    %<UpperLimit>
      | MIN = %<LowerLimit>
  Selector : Selector  InputPortWidth=3  IndexOptions=Index vector (dialog)  Indices=3  OutputSizes=1
  Selector1 : Selector  InputPortWidth=3  IndexOptions=Index vector (dialog)  Indices=[1 2]  OutputSizes=1
  Unit Delay : UnitDelay  SampleTime=0.01  HasFrameUpgradeWarning=on
  Unit Delay1 : UnitDelay  SampleTime=0.01  HasFrameUpgradeWarning=on
  ZXY_LIMITED : Scope  NumInputPorts=3
  prefilter : Subsystem  Commented=on  mask(Derivative Estimation){wn=2*pi*0.5, p=1}
      mask prompts: wn "Natural frequency, wn (rad/sec)"; p "Damping ratio, p"
      mask help:
      | A simple derivative estimator using a 2nd order representation between input and output.
      |
      | The integrators use a discrete FORWARd Euler rule, and a sample time needs to be specified.
      mask init:
      | str1 = sprintf('wn = %.2f', wn);
      | str2 = sprintf('p  = %.2f', p);
      | %str3 = sprintf('dt = %.2f', dt);
      | %str = char(str1,str2,str3);
      | %str3 = sprintf('dt = %.2f', dt);
      | str = char(str1,str2);
      mask Display: disp(str)
  XYZ : Outport  VectorParamsAs1DForOutWhenUnconnected=off
  CMD_BUS : Outport  Port=2  VectorParamsAs1DForOutWhenUnconnected=off
  wires:
  Selector1/1 -> Demux1/1, Unit Delay1/1
  Demux/1 -> Rate Limiter1/1
  Demux/2 -> Rate Limiter2/1
  Saturation1/1 -> [X]
  Saturation2/1 -> [Y]
  Mux4/1 -> Reshape/1
  Selector/1 -> Mux1/1, Unit Delay/1
  Rate Limiter/1 -> Saturation/1
  Unit Delay/1 -> Rate Limiter/1
  Unit Delay1/1 -> Demux/1
  Rate Limiter1/1 -> Saturation1/1
  Rate Limiter2/1 -> Saturation2/1
  [X] -> Mux4/1
  [Y] -> Mux4/2
  [Z] -> Mux4/3
  Saturation/1 -> [Z]
  [Z] -> Mux1/2
  [Y] -> Mux3/2
  Demux1/1 -> Mux2/1
  Demux1/2 -> Mux3/1
  [X] -> Mux2/2
  Mux1/1 -> ZXY_LIMITED/1  "Z"
  Mux2/1 -> ZXY_LIMITED/2  "X"
  Mux3/1 -> ZXY_LIMITED/3  "Y"
  Bus Creator/1 -> CMD_BUS/1
  [Y] -> Bus Creator/2  "Y"
  [X] -> Bus Creator/1  "X"
  [Z] -> Bus Creator/3  "Z"
  Reshape/1 -> XYZ/1
  XYZ_in/1 -> Selector1/1, Selector/1

== system bh_SM_quad_and_PEND_ORIG/a_circle1 ==
  Clock : Clock
  Clock1 : Clock
  Constant4 : Constant  Value=0  VectorParams1D=off
  Constant5 : Constant  Value=20  VectorParams1D=off
  Constant6 : Constant  Value=2  VectorParams1D=off
  Constant7 : Constant  VectorParams1D=off
  Constant8 : Constant  Value=0.05  VectorParams1D=off
  MATLAB Function : MATLAB Function  TreatAsAtomicUnit=on
  Mux1 : Mux  Inputs=3
  Reshape1 : Reshape  OutputDimensionality=Column vector (2-D)
  Reshape2 : Reshape  OutputDimensionality=Column vector (2-D)
  Signal Builder1 : Subsystem  Tag=STV Subsys  LoadFcn=sigbuilder_block('load');  StartFcn=sigbuilder_block('start');  StopFcn=sigbuilder_block('stop');  ClipboardFcn=sigbuilder_block('clipboard');  mask(Sigbuilder block){tuvar=[0:10]}
      mask help: Simulink:masks:SigbuilderBlock_MD
      mask init:
      | if ~strcmp(get_param(bdroot(gcbh),'SimulationStatus'),'stopped') tuvar = sigbuilder_block('maskInit'); end
      settings: CopyFcn=sigbuilder_block('copy');  DeleteFcn=sigbuilder_block('delete');  ModelCloseFcn=sigbuilder_block('modelClose');  PreSaveFcn=sigbuilder_block('preSave');  PauseFcn=sigbuilder_block('pause');  ContinueFcn=sigbuilder_block('continue');  NameChangeFcn=sigbuilder_block('namechange');  OpenFcn=sigbuilder_block('open',[437.6 199.2 550.4 400 ]);  CloseFcn=sigbuilder_block('close');
      mask Display: plot(0, 0, 100, 100,[2, 2, 32, 32, 2], [68, 8, 8, 68, 68],[32, 2], [38, 38], [32, 19, 2],[53, 60, 44], [32, 17, 17, 2],[16, 16, 31, 31]);txt = getActiveGroup(gcbh);text(2, 100, txt,'verticalAlignment', 'top');
  Subsystem : Subsystem
  Switch : Switch  Criteria=u2 > Threshold  Threshold=20
  Out1 : Outport  VectorParamsAs1DForOutWhenUnconnected=off
  wires:
  Switch/1 -> Out1/1
  MATLAB Function/1(XYZ) -> Reshape2/1
  Constant6/1 -> MATLAB Function/3(RADIUS)
  Constant7/1 -> MATLAB Function/4(ztgt)
  Subsystem/1(w_rad_psec) -> MATLAB Function/5(w)
  Constant5/1 -> MATLAB Function/2(t_to_start)
  Reshape1/1 -> Switch/3
  Constant4/1 -> Mux1/2
  Signal Builder1/1(Signal 1) -> Mux1/1
  Signal Builder1/2(Signal 2) -> Mux1/3
  Mux1/1 -> Reshape1/1
  Clock/1 -> Switch/2
  Clock1/1 -> MATLAB Function/1(t_clock)
  Constant8/1 -> Subsystem/1(RPS)
  Reshape2/1 -> Switch/1

== system bh_SM_quad_and_PEND_ORIG/CONT_SYS W_MOT_CMDS2/PRE_FILTERS ==
  w_in : Inport
  Demux : Demux
  Mux : Mux
  Reshape2 : Reshape  OutputDimensionality=Column vector (2-D)
  Terminator{,1..3} (4 alike) : Terminator
  prefilter : Subsystem  mask(Derivative Estimation){wn=2*pi*5, p=1}
      mask prompts: wn "Natural frequency, wn (rad/sec)"; p "Damping ratio, p"
      mask help:
      | A simple derivative estimator using a 2nd order representation between input and output.
      |
      | The integrators use a discrete FORWARd Euler rule, and a sample time needs to be specified.
      mask init:
      | str1 = sprintf('wn = %.2f', wn);
      | str2 = sprintf('p  = %.2f', p);
      | %str3 = sprintf('dt = %.2f', dt);
      | %str = char(str1,str2,str3);
      | %str3 = sprintf('dt = %.2f', dt);
      | str = char(str1,str2);
      mask Display: disp(str)
  prefilter1 : Subsystem  mask(Derivative Estimation){wn=2*pi*5, p=1}
      mask prompts: wn "Natural frequency, wn (rad/sec)"; p "Damping ratio, p"
      mask help:
      | A simple derivative estimator using a 2nd order representation between input and output.
      |
      | The integrators use a discrete FORWARd Euler rule, and a sample time needs to be specified.
      mask init:
      | str1 = sprintf('wn = %.2f', wn);
      | str2 = sprintf('p  = %.2f', p);
      | %str3 = sprintf('dt = %.2f', dt);
      | %str = char(str1,str2,str3);
      | %str3 = sprintf('dt = %.2f', dt);
      | str = char(str1,str2);
      mask Display: disp(str)
  prefilter2 : Subsystem  mask(Derivative Estimation){wn=2*pi*5, p=1}
      mask prompts: wn "Natural frequency, wn (rad/sec)"; p "Damping ratio, p"
      mask help:
      | A simple derivative estimator using a 2nd order representation between input and output.
      |
      | The integrators use a discrete FORWARd Euler rule, and a sample time needs to be specified.
      mask init:
      | str1 = sprintf('wn = %.2f', wn);
      | str2 = sprintf('p  = %.2f', p);
      | %str3 = sprintf('dt = %.2f', dt);
      | %str = char(str1,str2,str3);
      | %str3 = sprintf('dt = %.2f', dt);
      | str = char(str1,str2);
      mask Display: disp(str)
  prefilter3 : Subsystem  mask(Derivative Estimation){wn=2*pi*5, p=1}
      mask prompts: wn "Natural frequency, wn (rad/sec)"; p "Damping ratio, p"
      mask help:
      | A simple derivative estimator using a 2nd order representation between input and output.
      |
      | The integrators use a discrete FORWARd Euler rule, and a sample time needs to be specified.
      mask init:
      | str1 = sprintf('wn = %.2f', wn);
      | str2 = sprintf('p  = %.2f', p);
      | %str3 = sprintf('dt = %.2f', dt);
      | %str = char(str1,str2,str3);
      | %str3 = sprintf('dt = %.2f', dt);
      | str = char(str1,str2);
      mask Display: disp(str)
  w CMD vs Actual : Scope  NumInputPorts=4
  w_MUX : Subsystem
  w : Outport  VectorParamsAs1DForOutWhenUnconnected=off
  wires:
  prefilter1/2(U_DOT) -> Terminator1/1
  prefilter/2(U_DOT) -> Terminator/1
  prefilter2/2(U_DOT) -> Terminator2/1
  prefilter3/2(U_DOT) -> Terminator3/1
  w_in/1 -> [W_CMD], Demux/1
  Demux/1 -> prefilter/1(U)
  Demux/2 -> prefilter1/1(U)
  Demux/3 -> prefilter2/1(U)
  Demux/4 -> prefilter3/1(U)
  prefilter/1(U_filt) -> Mux/1
  prefilter1/1(U_filt) -> Mux/2
  prefilter2/1(U_filt) -> Mux/3
  prefilter3/1(U_filt) -> Mux/4
  Mux/1 -> Reshape2/1
  Reshape2/1 -> w_MUX/2(W), w/1
  w_MUX/3(w3) -> w CMD vs Actual/3
  w_MUX/2(w2) -> w CMD vs Actual/2
  w_MUX/4(w4) -> w CMD vs Actual/4
  [W_CMD] -> w_MUX/1(W_CMD)
  w_MUX/1(w1) -> w CMD vs Actual/1

== system bh_SM_quad_and_PEND_ORIG/CONT_SYS W_MOT_CMDS2/SIGN_CONVENTIONS ==

== system bh_SM_quad_and_PEND_ORIG/CONT_SYS W_MOT_CMDS2/W2_checker ==
  w2_CMD : Inport
  Assertion{,1..3} (4 alike) : Assertion
  Compare To Constant : simulink/Logic and Bit Operations/Compare To Constant  relop=>=  const=0  OutDataTypeStr=boolean
  Demux : Demux
  w2 : Outport  VectorParamsAs1DForOutWhenUnconnected=off
  wires:
  w2_CMD/1 -> w2/1, Compare To Constant/1
  Compare To Constant/1 -> Demux/1
  Demux/1 -> Assertion/1
  Demux/4 -> Assertion3/1
  Demux/3 -> Assertion2/1
  Demux/2 -> Assertion1/1

== system bh_SM_quad_and_PEND_ORIG/EYES_PROP_and_VEH/THRUST_FUSE ==
  REF : Inport
  p1_b : Inport  Port=2
  p2_b : Inport  Port=3
  p3_b : Inport  Port=4
  p4_b : Inport  Port=5
  Bus Selector{,1..3} (4 alike) : BusSelector  OutputSignals=Thrust_on_veh
  Mux{,1..3} (4 alike) : Mux  Inputs=2
  Selector : Selector  InputPortWidth=4  IndexOptions=Index vector (dialog)  Indices=1  OutputSizes=1
  Selector1 : Selector  InputPortWidth=4  IndexOptions=Index vector (dialog)  Indices=2  OutputSizes=1
  Selector2 : Selector  InputPortWidth=4  IndexOptions=Index vector (dialog)  Indices=3  OutputSizes=1
  Selector3 : Selector  InputPortWidth=4  IndexOptions=Index vector (dialog)  Indices=4  OutputSizes=1
  Out1 : Outport  VectorParamsAs1DForOutWhenUnconnected=off
  Out2 : Outport  Port=2  VectorParamsAs1DForOutWhenUnconnected=off
  Out3 : Outport  Port=3  VectorParamsAs1DForOutWhenUnconnected=off
  Out4 : Outport  Port=4  VectorParamsAs1DForOutWhenUnconnected=off
  wires:
  Mux/1 -> Out4/1
  Mux1/1 -> Out3/1
  Mux2/1 -> Out2/1
  Mux3/1 -> Out1/1
  p1_b/1 -> Bus Selector/1
  Bus Selector/1 -> Mux3/2  "<Thrust_on_veh>"
  Selector/1 -> Mux3/1
  Selector1/1 -> Mux2/1
  Selector2/1 -> Mux1/1
  Selector3/1 -> Mux/1
  REF/1 -> Selector3/1, Selector2/1, Selector1/1, Selector/1
  p2_b/1 -> Bus Selector1/1
  Bus Selector1/1 -> Mux2/2  "<Thrust_on_veh>"
  p3_b/1 -> Bus Selector2/1
  Bus Selector2/1 -> Mux1/2  "<Thrust_on_veh>"
  p4_b/1 -> Bus Selector3/1
  Bus Selector3/1 -> Mux/2  "<Thrust_on_veh>"

== system bh_SM_quad_and_PEND_ORIG/EYES_PROP_and_VEH/TQ_FUSE ==
  REF : Inport
  p1_b : Inport  Port=2
  p2_b : Inport  Port=3
  p3_b : Inport  Port=4
  p4_b : Inport  Port=5
  Bus Selector{,1..3} (4 alike) : BusSelector  OutputSignals=Torque_on_veh
  Mux{,1..3} (4 alike) : Mux  Inputs=2
  Selector : Selector  InputPortWidth=4  IndexOptions=Index vector (dialog)  Indices=1  OutputSizes=1
  Selector1 : Selector  InputPortWidth=4  IndexOptions=Index vector (dialog)  Indices=2  OutputSizes=1
  Selector2 : Selector  InputPortWidth=4  IndexOptions=Index vector (dialog)  Indices=3  OutputSizes=1
  Selector3 : Selector  InputPortWidth=4  IndexOptions=Index vector (dialog)  Indices=4  OutputSizes=1
  Out1 : Outport  VectorParamsAs1DForOutWhenUnconnected=off
  Out2 : Outport  Port=2  VectorParamsAs1DForOutWhenUnconnected=off
  Out3 : Outport  Port=3  VectorParamsAs1DForOutWhenUnconnected=off
  Out4 : Outport  Port=4  VectorParamsAs1DForOutWhenUnconnected=off
  wires:
  Mux/1 -> Out4/1
  Mux1/1 -> Out3/1
  Mux2/1 -> Out2/1
  Mux3/1 -> Out1/1
  p1_b/1 -> Bus Selector/1
  Bus Selector/1 -> Mux3/2  "<Torque_on_veh>"
  Selector/1 -> Mux3/1
  Selector1/1 -> Mux2/1
  Selector2/1 -> Mux1/1
  Selector3/1 -> Mux/1
  REF/1 -> Selector3/1, Selector2/1, Selector1/1, Selector/1
  p2_b/1 -> Bus Selector1/1
  Bus Selector1/1 -> Mux2/2  "<Torque_on_veh>"
  p3_b/1 -> Bus Selector2/1
  Bus Selector2/1 -> Mux1/2  "<Torque_on_veh>"
  p4_b/1 -> Bus Selector3/1
  Bus Selector3/1 -> Mux/2  "<Torque_on_veh>"

== system bh_SM_quad_and_PEND_ORIG/EYES_PROP_and_VEH/w_FUSE ==
  REF : Inport
  p1_b : Inport  Port=2
  p2_b : Inport  Port=3
  p3_b : Inport  Port=4
  p4_b : Inport  Port=5
  Bus Selector{,1..3} (4 alike) : BusSelector  OutputSignals=w_prop
  Mux{,1..3} (4 alike) : Mux  Inputs=2
  Selector : Selector  InputPortWidth=4  IndexOptions=Index vector (dialog)  Indices=1  OutputSizes=1
  Selector1 : Selector  InputPortWidth=4  IndexOptions=Index vector (dialog)  Indices=2  OutputSizes=1
  Selector2 : Selector  InputPortWidth=4  IndexOptions=Index vector (dialog)  Indices=3  OutputSizes=1
  Selector3 : Selector  InputPortWidth=4  IndexOptions=Index vector (dialog)  Indices=4  OutputSizes=1
  Out1 : Outport  VectorParamsAs1DForOutWhenUnconnected=off
  Out2 : Outport  Port=2  VectorParamsAs1DForOutWhenUnconnected=off
  Out3 : Outport  Port=3  VectorParamsAs1DForOutWhenUnconnected=off
  Out4 : Outport  Port=4  VectorParamsAs1DForOutWhenUnconnected=off
  wires:
  Mux/1 -> Out4/1
  Mux1/1 -> Out3/1
  Mux2/1 -> Out2/1
  Mux3/1 -> Out1/1
  p1_b/1 -> Bus Selector/1
  Bus Selector/1 -> Mux3/2  "<w_prop>"
  Selector/1 -> Mux3/1
  Selector1/1 -> Mux2/1
  Selector2/1 -> Mux1/1
  Selector3/1 -> Mux/1
  REF/1 -> Selector3/1, Selector2/1, Selector1/1, Selector/1
  Bus Selector1/1 -> Mux2/2  "<w_prop>"
  p2_b/1 -> Bus Selector1/1
  Bus Selector2/1 -> Mux1/2  "<w_prop>"
  p3_b/1 -> Bus Selector2/1
  Bus Selector3/1 -> Mux/2  "<w_prop>"
  p4_b/1 -> Bus Selector3/1

== system bh_SM_quad_and_PEND_ORIG/MODEL_SYS/SIGN_CONVENTIONS ==

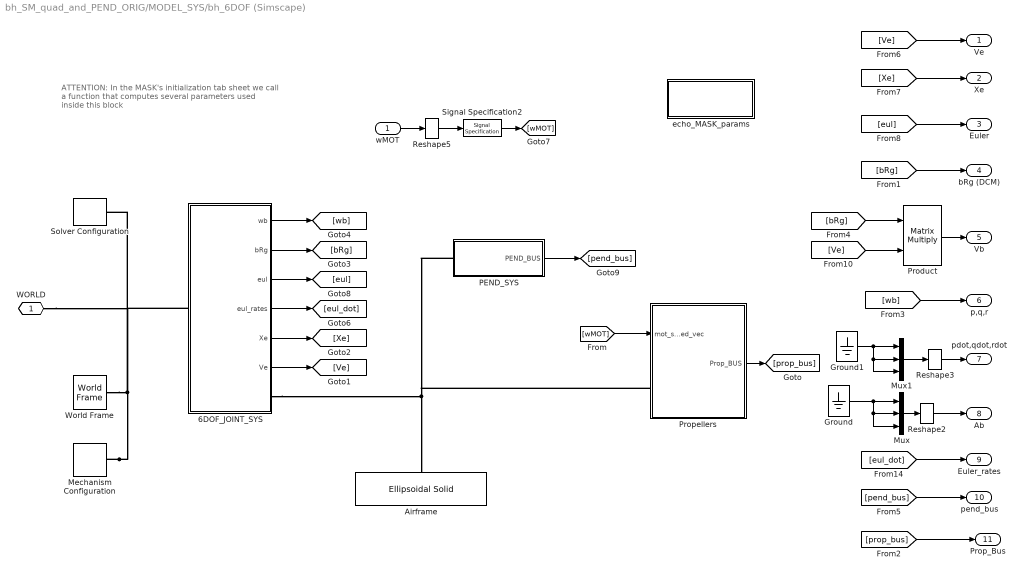
== system bh_SM_quad_and_PEND_ORIG/MODEL_SYS/bh_6DOF (Simscape) ==
  note: ATTENTION:
      | In the MASK's initialization tab sheet
      | we call a function that computes several parameters
      | used inside this block
  wMOT : Inport
  6DOF_JOINT_SYS : Subsystem
  Airframe : sm_lib/Body Elements/Ellipsoidal Solid  GraphicAmbientColor=[0.15 0.15 0.15 1.0]  BasedOnType=Density  CenterOfMass=[0 0 0]  CenterOfMassUnits=m  GraphicDiffuseColor=[0.5 0.5 0.5]  Density=1000  DensityUnits=kg/(m^3)  DoExposeReferenceFrame=on  EllipsoidRadii=[prop_CG_L, prop_CG_L, prop_CG_L/10]  EllipsoidRadiiUnits=m  GraphicEmissiveColor=[0.0 0.0 0.0 1.0]  ExportEntireGeometry=off  SerializedFrames=<Frames/>  MarkerShape=Sphere  MarkerSize=10  GraphicType=FromGeometry  InertiaType=Custom  Mass=air_mass_0  MassUnits=kg  MomentsOfInertia=Iair_xx_yy_zz  MomentsOfInertiaUnits=kg*m^2  GraphicOpacity=1.0  ProductsOfInertia=Iair_yz_zx_xy  ProductsOfInertiaUnits=kg*m^2  GraphicShininess=75  GraphicSpecularColor=[0.5 0.5 0.5 1.0]  GraphicVisPropType=SimpleVisualProperties
      settings: SourceProductBaseCode=MS
      settings: AttributesFormatString=|
      | %<Mass>
      | %<MomentsOfInertia>
      | %<ProductsOfInertia>
  Ground : Ground
  Ground1 : Ground
  Mechanism Configuration : sm_lib/Utilities/Mechanism Configuration  UniformGravity=Constant  GravityVector=[0, 0, -g_const]  GravityUnits=m/s^2  LinearizationDelta=0.001
  Mux : Mux  Inputs=3
  Mux1 : Mux  Inputs=3
  PEND_SYS : Subsystem
  Product : Product  Multiplication=Matrix(*)
  Propellers : Subsystem
  Reshape2 : Reshape  OutputDimensionality=Column vector (2-D)
  Reshape3 : Reshape  OutputDimensionality=Column vector (2-D)
  Reshape5 : Reshape  OutputDimensionality=Column vector (2-D)
  Signal Specification2 : SignalSpecification  Dimensions=[4,1]
  Solver Configuration : nesl_utility/Solver Configuration  PhysicalDomain=network_engine_domain  SubClassName=solver  LeftPortType=input  RightPortType=generic  Tones=[]  Harmonics=[]  SimulateNoise=off  Profile=off  UseLocalSampling=off  EnableSwitchedLinearOptims=on  FrequencyDomain=off  UseCCode=off  RelTol=0.001  AbsTol=1e-06  MinStep=1e-09  ToWorkspace=off  RevertToSquareIcSolve=off  NumHomotopyIterations=100  PhasorMode=off  PhasorModeNumHarmonics=1  DoDC=off  ResidualTolerance=1e-09  UseLocalSolver=off  LocalSolverChoice=NE_BACKWARD_EULER_ADVANCER  LocalSolverSampleTime=0.001  DoFixedCost=off  MaxNonlinIter=3  MaxModeIter=2  LinearAlgebra=Sparse  EquationFormulation=NE_TIME_EF  DelaysMemoryBudget=1024  AutomaticFiltering=on  FilteringTimeConstant=0.001  PartitionStorageMethod=AS_NEEDED  PartitionMemoryBudget=1024  PartitionMethod=FAST
  World Frame : sm_lib/Frames and Transforms/World Frame
  echo_MASK_params : Subsystem
  WORLD : PMIOPort  Side=Left
  Ve : Outport  VectorParamsAs1DForOutWhenUnconnected=off
  Xe : Outport  Port=2  VectorParamsAs1DForOutWhenUnconnected=off
  Euler : Outport  Port=3  VectorParamsAs1DForOutWhenUnconnected=off
  bRg (DCM) : Outport  Port=4  VectorParamsAs1DForOutWhenUnconnected=off
  Vb : Outport  Port=5  VectorParamsAs1DForOutWhenUnconnected=off
  p,q,r : Outport  Port=6  VectorParamsAs1DForOutWhenUnconnected=off
  pdot,qdot,rdot : Outport  Port=7  VectorParamsAs1DForOutWhenUnconnected=off
  Ab : Outport  Port=8  VectorParamsAs1DForOutWhenUnconnected=off
  Euler_rates : Outport  Port=9  VectorParamsAs1DForOutWhenUnconnected=off
  pend_bus : Outport  Port=10  VectorParamsAs1DForOutWhenUnconnected=off
  Prop_Bus : Outport  Port=11  VectorParamsAs1DForOutWhenUnconnected=off
  wires:
  [Ve] -> Ve/1
  [Xe] -> Xe/1
  [eul] -> Euler/1
  [bRg] -> bRg (DCM)/1
  Mux/1 -> Reshape2/1
  Reshape2/1 -> Ab/1
  Ground/1 -> Mux/2, Mux/3, Mux/1
  Product/1 -> Vb/1
  [wb] -> p,q,r/1
  [eul_dot] -> Euler_rates/1
  Ground1/1 -> Mux1/2, Mux1/3, Mux1/1
  Reshape3/1 -> pdot,qdot,rdot/1
  Mux1/1 -> Reshape3/1
  wMOT/1 -> Reshape5/1
  Reshape5/1 -> Signal Specification2/1
  Signal Specification2/1 -> [wMOT]
  [wMOT] -> Propellers/1(mot_speed_vec)
  6DOF_JOINT_SYS/2(bRg) -> [bRg]
  6DOF_JOINT_SYS/5(Xe) -> [Xe]
  6DOF_JOINT_SYS/6(Ve) -> [Ve]
  6DOF_JOINT_SYS/1(wb) -> [wb]
  [Ve] -> Product/2
  [bRg] -> Product/1
  6DOF_JOINT_SYS/4(eul_rates) -> [eul_dot]
  6DOF_JOINT_SYS/3(eul) -> [eul]
  PEND_SYS/1(PEND_BUS) -> [pend_bus]
  [pend_bus] -> pend_bus/1
  Propellers/1(Prop_BUS) -> [prop_bus]
  [prop_bus] -> Prop_Bus/1
  connections:
  Mechanism Configuration/RConn1 -- WORLD/RConn1 -- 6DOF_JOINT_SYS/LConn1 -- Solver Configuration/RConn1 -- World Frame/RConn1
  6DOF_JOINT_SYS/RConn1 -- Propellers/LConn1 -- PEND_SYS/LConn1 -- Airframe/RConn1

== system bh_SM_quad_and_PEND_ORIG/SAR/XYZ_CMDS ==
  Demux : Demux  Tag=STV Demux  Outputs=3
      settings: DisplayOption=none
  FromWs : FromWorkspace  Tag=STV FromWs  VariableName=tuvar
      SigBuilderData=|
      | common.afterFinalStr = 'Extrapolate'
      | common.sampleTime = 0
      | dataSet(1).timeRange = [0 200]
      | dataSet(1).name = 'small_steps'
      | dataSet(2).timeRange = [0 200]
      | dataSet(2).name = 'zStairs_xyConstVEL'
      | dataSet(3).timeRange = [0 500]
      | dataSet(3).name = 'sineWaves'
      | dataSet(4).timeRange = [0 200]
      | dataSet(4).name = 'ZERO'
      | dataSet(5).timeRange = [0 200]
      | dataSet(5).name = 'SEARCH_P1'
      | sbobj.Name = 'Signal Builder'
      | sbobj.Groups(1).Name = 'small_steps'
      | sbobj.Groups(1).Signals(1).Name = 'Z'
      | sbobj.Groups(1).Signals(1).XData = [0 10 10.000001 20 20.000001 30 30.000001 55 200]
      | sbobj.Groups(1).Signals(1).YData = [0 0 2 2 2 2 2 2 2]
      | sbobj.Groups(1).Signals(2).Name = 'X'
      | sbobj.Groups(1).Signals(2).XData = [0 10 10.000001 20 20.000001 30 30.000001 55 200]
      | sbobj.Groups(1).Signals(2).YData = [0 0 0 0 3 3 3 3 3]
      | sbobj.Groups(1).Signals(3).Name = 'Y'
      | sbobj.Groups(1).Signals(3).XData = [0 10 10.000001 20 20.000001 30 30.000001 55 200]
      | sbobj.Groups(1).Signals(3).YData = [0 0 0 0 0 0 1 1 1]
      | sbobj.Groups(1).TimeRange = [0 200]
      | sbobj.Groups(2).Name = 'zStairs_xyConstVEL'
      | sbobj.Groups(2).Signals(1).Name = 'Z'
      | sbobj.Groups(2).Signals(1).XData = [0 10 10.000001 20 20.000001 30 30.000001 40 40.000001 55 200]
      | sbobj.Groups(2).Signals(1).YData = [0 0 1 1 2 2 1 1 0 0 0]
      | sbobj.Groups(2).Signals(2).Name = 'X'
      | sbobj.Groups(2).Signals(2).XData = [0 10 10.000001 20 20.000001 30 30.000001 40 40.000001 55 200]
      | sbobj.Groups(2).Signals(2).YData = [0 1 1.0000001 2 2.0000001 3 3.0000001 4 4.0000001 5.5 20]
      | sbobj.Groups(2).Signals(3).Name = 'Y'
      | sbobj.Groups(2).Signals(3).XData = [0 10 10.000001 20 20.000001 30 30.000001 40 40.000001 55 200]
      | sbobj.Groups(2).Signals(3).YData = [0 0.5 0.50000005 1 1.00000005 1.5 1.50000005 2 2.00000005 2.75 10]
      | sbobj.Groups(2).TimeRange = [0 200]
      | sbobj.Groups(3).Name = 'sineWaves'
      | sbobj.Groups(3).Signals(1).Name = 'Z'
      | sbobj.Groups(3).Signals(1).XData = [0 0.1 0.2 0.3 0.4 0.5 0.6 0.7 0.8 0.9 1 1.1 ... (5001 elements, 1x5001)]
      | sbobj.Groups(3).Signals(1).YData = [0 0.0314107325553 0.0627904665622 0.0941082340641 0.125333128258 0.156434333994 0.18738115819 0.218143060119 0.248689681547 0.278990876699 0.309016742004 0.338737645607 ... (5001 elements, 1x5001)]
      | sbobj.Groups(3).Signals(2).Name = 'X'
      | sbobj.Groups(3).Signals(2).XData = [0 0.1 0.2 0.3 0.4 0.5 0.6 0.7 0.8 0.9 1 1.1 ... (5001 elements, 1x5001)]
      | sbobj.Groups(3).Signals(2).YData = [0 0.01 0.02 0.03 0.04 0.05 0.06 0.07 0.08 0.09 0.1 0.11 ... (5001 elements, 1x5001)]
      | sbobj.Groups(3).Signals(3).Name = 'Y'
      | sbobj.Groups(3).Signals(3).XData = [0 0.1 0.2 0.3 0.4 0.5 0.6 0.7 0.8 0.9 1 1.1 ... (5001 elements, 1x5001)]
      | sbobj.Groups(3).Signals(3).YData = [0 0.0157073040455 0.0314107325553 0.04710641095 0.0627904665622 0.0784590295926 0.0941082340641 0.109734218776 0.125333128258 0.140901113717 0.156434333994 0.171928956505 ... (5001 elements, 1x5001)]
      | sbobj.Groups(3).TimeRange = [0 500]
      | sbobj.Groups(4).Name = 'ZERO'
      | sbobj.Groups(4).Signals(1).Name = 'Z'
      | sbobj.Groups(4).Signals(1).XData = [0 200]
      | sbobj.Groups(4).Signals(1).YData = [0 0]
      | sbobj.Groups(4).Signals(2).Name = 'X'
      | sbobj.Groups(4).Signals(2).XData = [0 200]
      | sbobj.Groups(4).Signals(2).YData = [0 0]
      | sbobj.Groups(4).Signals(3).Name = 'Y'
      | sbobj.Groups(4).Signals(3).XData = [0 200]
      | sbobj.Groups(4).Signals(3).YData = [0 0]
      | sbobj.Groups(4).TimeRange = [0 200]
      | sbobj.Groups(5).Name = 'SEARCH_P1'
      | sbobj.Groups(5).Signals(1).Name = 'Z'
      | sbobj.Groups(5).Signals(1).XData = [0 7 27 32 52 57 77 82 102 107 127 132 157 187 200]
      | sbobj.Groups(5).Signals(1).YData = [0 5 5 5 5 5 5 5 5 5 5 5 5 0 0]
      | sbobj.Groups(5).Signals(2).Name = 'X'
      | sbobj.Groups(5).Signals(2).XData = [0 7 27 32 52 57 77 82 102 107 127 132 157 187 200]
      | sbobj.Groups(5).Signals(2).YData = [0 5 25 25 5 5 25 25 5 5 25 25 0 0 0]
      | sbobj.Groups(5).Signals(3).Name = 'Y'
      | sbobj.Groups(5).Signals(3).XData = [0 7 27 32 52 57 77 82 102 107 127 132 157 187 200]
      | sbobj.Groups(5).Signals(3).YData = [0 5 5 10 10 15 15 20 20 25 25 30 30 0 0]
      | sbobj.Groups(5).TimeRange = [0 200]
  Z : Outport  VectorParamsAs1DForOutWhenUnconnected=off
  X : Outport  Tag=STV Outport  Port=2  VectorParamsAs1DForOutWhenUnconnected=off
  Y : Outport  Tag=STV Outport  Port=3  VectorParamsAs1DForOutWhenUnconnected=off
  wires:
  Demux/1 -> Z/1
  FromWs/1 -> Demux/1
  Demux/2 -> X/1
  Demux/3 -> Y/1

== system bh_SM_quad_and_PEND_ORIG/XYZ CMD_LIMITS/prefilter ==
  note: Y = U *     wn^2/( s^2 + 2*p*wn*s + wn^2)
      | Y*( s^2 + 2*p*wn*s + wn^2) = U * wn^2
      |
      | y'' + y'*2*p*wn + y*wn^2 = U*wn^2
  U : Inport
  Gain : Gain  Gain=2*p*wn
  Gain1 : Gain  Gain=wn^2
  Gain2 : Gain  Gain=wn^2
  Integrator : Integrator
  Integrator1 : Integrator
  Sum : Sum  Inputs=|+--
  U_filt : Outport  VectorParamsAs1DForOutWhenUnconnected=off
  U_DOT : Outport  Port=2  VectorParamsAs1DForOutWhenUnconnected=off
  wires:
  Integrator/1 -> Integrator1/1, [Y_DOT], Gain/1  "y_dot"
  Sum/1 -> Integrator/1  "y_dot_dot"
  Integrator1/1 -> Gain1/1, U_filt/1  "y"
  U/1 -> Gain2/1
  Gain2/1 -> Sum/1
  Gain/1 -> Sum/3
  Gain1/1 -> Sum/2
  [Y_DOT] -> U_DOT/1

== system bh_SM_quad_and_PEND_ORIG/a_circle1/Signal Builder1 ==
  Demux : Demux  Tag=STV Demux  Outputs=2
      settings: DisplayOption=none
  FromWs : FromWorkspace  Tag=STV FromWs  VariableName=tuvar
      SigBuilderData=|
      | common.afterFinalStr = 'Extrapolate'
      | common.sampleTime = 0
      | dataSet.timeRange = [0 22]
      | dataSet.name = 'Group 1'
      | sbobj.Groups.Name = 'Group 1'
      | sbobj.Groups.Signals(1).Name = 'Signal 1'
      | sbobj.Groups.Signals(1).XData = [0 7.95 7.95 22]
      | sbobj.Groups.Signals(1).YData = [0 0 1.99 1.98]
      | sbobj.Groups.Signals(2).Name = 'Signal 2'
      | sbobj.Groups.Signals(2).XData = [0 12 16 22]
      | sbobj.Groups.Signals(2).YData = [0 0 1 1]
      | sbobj.Groups.TimeRange = [0 22]
  Signal 1 : Outport  Tag=STV Outport  VectorParamsAs1DForOutWhenUnconnected=off
  Signal 2 : Outport  Tag=STV Outport  Port=2  VectorParamsAs1DForOutWhenUnconnected=off
  wires:
  Demux/1 -> Signal 1/1
  FromWs/1 -> Demux/1
  Demux/2 -> Signal 2/1

== system bh_SM_quad_and_PEND_ORIG/a_circle1/Subsystem ==
  RPS : Inport
  Constant : Constant  Value=2*pi
  Product : Product  Inputs=**
  w_rad_psec : Outport  VectorParamsAs1DForOutWhenUnconnected=off
  wires:
  Constant/1 -> Product/2
  RPS/1 -> Product/1
  Product/1 -> w_rad_psec/1

== system bh_SM_quad_and_PEND_ORIG/CONT_SYS W_MOT_CMDS2/PRE_FILTERS/prefilter ==
  note: Y = U *     wn^2/( s^2 + 2*p*wn*s + wn^2)
      | Y*( s^2 + 2*p*wn*s + wn^2) = U * wn^2
      |
      | y'' + y'*2*p*wn + y*wn^2 = U*wn^2
  U : Inport
  Gain : Gain  Gain=2*p*wn
  Gain1 : Gain  Gain=wn^2
  Gain2 : Gain  Gain=wn^2
  Integrator : Integrator
  Integrator1 : Integrator
  Sum : Sum  Inputs=|+--
  U_filt : Outport  VectorParamsAs1DForOutWhenUnconnected=off
  U_DOT : Outport  Port=2  VectorParamsAs1DForOutWhenUnconnected=off
  wires:
  Integrator/1 -> Integrator1/1, [Y_DOT], Gain/1  "y_dot"
  Sum/1 -> Integrator/1  "y_dot_dot"
  Integrator1/1 -> Gain1/1, U_filt/1  "y"
  U/1 -> Gain2/1
  Gain2/1 -> Sum/1
  Gain/1 -> Sum/3
  Gain1/1 -> Sum/2
  [Y_DOT] -> U_DOT/1

== system bh_SM_quad_and_PEND_ORIG/CONT_SYS W_MOT_CMDS2/PRE_FILTERS/prefilter1 ==
  note: Y = U *     wn^2/( s^2 + 2*p*wn*s + wn^2)
      | Y*( s^2 + 2*p*wn*s + wn^2) = U * wn^2
      |
      | y'' + y'*2*p*wn + y*wn^2 = U*wn^2
  U : Inport
  Gain : Gain  Gain=2*p*wn
  Gain1 : Gain  Gain=wn^2
  Gain2 : Gain  Gain=wn^2
  Integrator : Integrator
  Integrator1 : Integrator
  Sum : Sum  Inputs=|+--
  U_filt : Outport  VectorParamsAs1DForOutWhenUnconnected=off
  U_DOT : Outport  Port=2  VectorParamsAs1DForOutWhenUnconnected=off
  wires:
  Integrator/1 -> Integrator1/1, [Y_DOT], Gain/1  "y_dot"
  Sum/1 -> Integrator/1  "y_dot_dot"
  Integrator1/1 -> Gain1/1, U_filt/1  "y"
  U/1 -> Gain2/1
  Gain2/1 -> Sum/1
  Gain/1 -> Sum/3
  Gain1/1 -> Sum/2
  [Y_DOT] -> U_DOT/1
